simulink model "main_model_mode8"  (R2026a)
settings: Solver=ode4  StopTime=30  FixedStep=1e-4
undefined symbols (not defined in the file or in its folder): dspblkCoreblockFVToolHelper, gcbh
libraries: simulink x12, dspstat3 x3

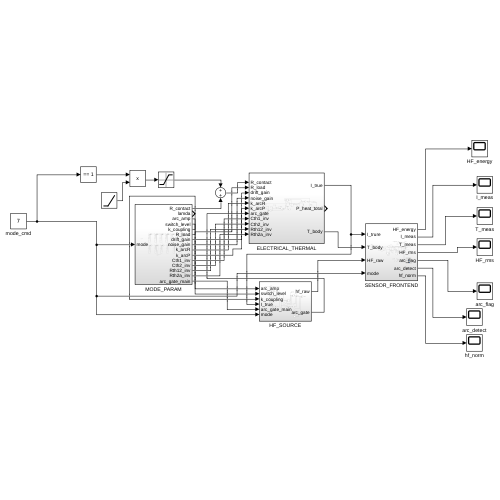
[thumbnail: Simulink's stored preview of the top-level diagram]
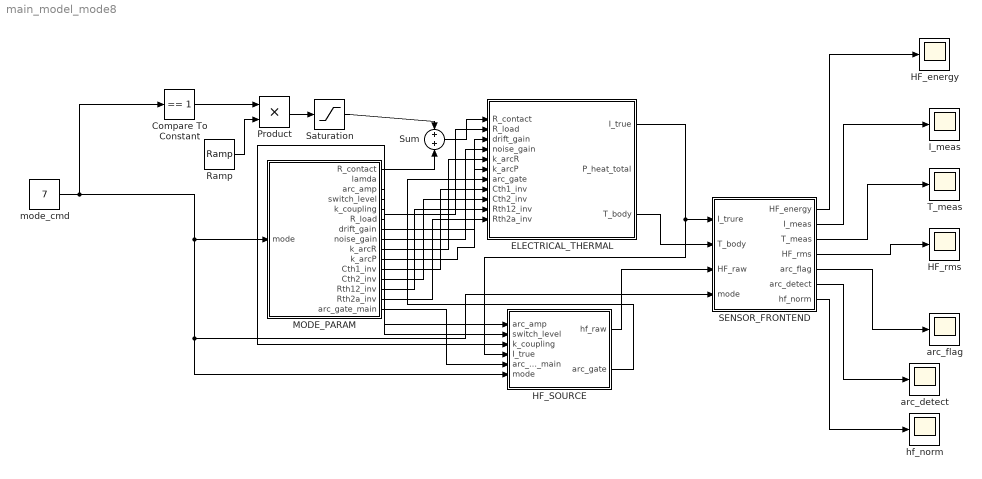
== system main_model_mode8 ==
  Compare To Constant : simulink/Logic and Bit Operations/Compare To Constant  relop===  const=1  OutDataTypeStr=boolean
  ELECTRICAL_THERMAL : Subsystem
  HF_SOURCE : Subsystem
  HF_energy : Scope
      settings: ActiveDisplayYMinimum=-510.38723335588418  ActiveDisplayYMaximum=4593.4851017280953
  HF_rms : Scope
      settings: ActiveDisplayYMinimum=-1  ActiveDisplayYMaximum=1  DataLoggingVariableName=ScopeData3
  I_meas : Scope
      settings: ActiveDisplayYMinimum=-209.09631630294618  ActiveDisplayYMaximum=207.20339945692962
  MODE_PARAM : Subsystem
  Product : Product
  Ramp : simulink/Sources/Ramp  slope=0.002  start=0  InitialOutput=0
  SENSOR_FRONTEND : Subsystem
  Saturation : Saturate  UpperLimit=0.05  LowerLimit=0
  Sum : Sum
  T_meas : Scope
      settings: ActiveDisplayYMinimum=-24.999999999999993  ActiveDisplayYMaximum=225  DataLoggingVariableName=ScopeData2
  arc_detect : Scope
      settings: ActiveDisplayYMinimum=-1  ActiveDisplayYMaximum=1  DataLoggingVariableName=ScopeData10
  arc_flag : Scope
      settings: ActiveDisplayYMinimum=-1  ActiveDisplayYMaximum=1  DataLoggingVariableName=ScopeData9
  hf_norm : Scope
      settings: ActiveDisplayYMinimum=-541.8103571547914  ActiveDisplayYMaximum=4968.8787163023626  DataLoggingVariableName=ScopeData11
  mode_cmd : Constant  Value=7
  wires:
  ELECTRICAL_THERMAL/1(I_true) -> HF_SOURCE/4(I_true), SENSOR_FRONTEND/1(I_trure)
  mode_cmd/1 -> HF_SOURCE/6(mode), SENSOR_FRONTEND/4(mode), MODE_PARAM/1(mode), Compare To Constant/1
  Compare To Constant/1 -> Product/1
  Ramp/1 -> Product/2
  Product/1 -> Saturation/1
  Saturation/1 -> Sum/1
  MODE_PARAM/1(R_contact) -> Sum/2
  Sum/1 -> ELECTRICAL_THERMAL/1(R_contact)
  SENSOR_FRONTEND/2(I_meas) -> I_meas/1
  SENSOR_FRONTEND/3(T_meas) -> T_meas/1
  SENSOR_FRONTEND/1(HF_energy) -> HF_energy/1
  SENSOR_FRONTEND/4(HF_rms) -> HF_rms/1
  MODE_PARAM/6(R_load) -> ELECTRICAL_THERMAL/2(R_load)
  MODE_PARAM/7(drift_gain) -> ELECTRICAL_THERMAL/3(drift_gain)
  MODE_PARAM/8(noise_gain) -> ELECTRICAL_THERMAL/4(noise_gain)
  MODE_PARAM/9(k_arcR) -> ELECTRICAL_THERMAL/5(k_arcR)
  MODE_PARAM/10(k_arcP) -> ELECTRICAL_THERMAL/6(k_arcP)
  MODE_PARAM/11(Cth1_inv) -> ELECTRICAL_THERMAL/8(Cth1_inv)
  MODE_PARAM/12(Cth2_inv) -> ELECTRICAL_THERMAL/9(Cth2_inv)
  MODE_PARAM/13(Rth12_inv) -> ELECTRICAL_THERMAL/10(Rth12_inv)
  MODE_PARAM/14(Rth2a_inv) -> ELECTRICAL_THERMAL/11(Rth2a_inv)
  ELECTRICAL_THERMAL/3(T_body) -> SENSOR_FRONTEND/2(T_body)
  HF_SOURCE/1(hf_raw) -> SENSOR_FRONTEND/3(HF_raw)
  MODE_PARAM/5(k_coupling) -> HF_SOURCE/3(k_coupling)
  MODE_PARAM/4(switch_level) -> HF_SOURCE/2(switch_level)
  MODE_PARAM/3(arc_amp) -> HF_SOURCE/1(arc_amp)
  HF_SOURCE/2(arc_gate) -> ELECTRICAL_THERMAL/7(arc_gate)
  MODE_PARAM/15(arc_gate_main) -> HF_SOURCE/5(arc_gate_main)
  SENSOR_FRONTEND/5(arc_flag) -> arc_flag/1
  SENSOR_FRONTEND/6(arc_detect) -> arc_detect/1
  SENSOR_FRONTEND/7(hf_norm) -> hf_norm/1

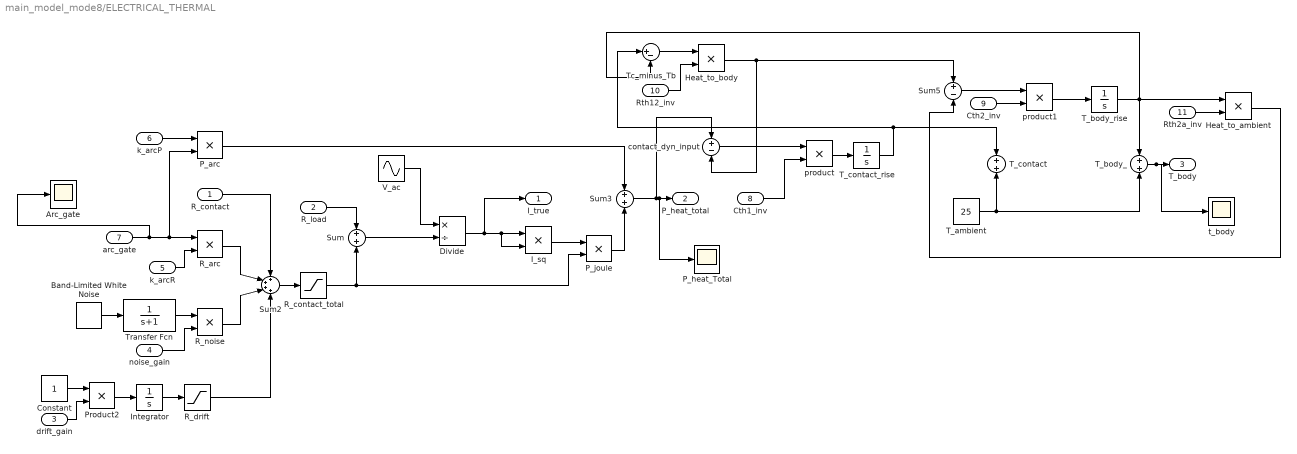
== system main_model_mode8/ELECTRICAL_THERMAL ==
  R_contact : Inport
  R_load : Inport  Port=2
  drift_gain : Inport  Port=3
  noise_gain : Inport  Port=4
  k_arcR : Inport  Port=5
  k_arcP : Inport  Port=6
  arc_gate : Inport  Port=7
  Cth1_inv : Inport  Port=8
  Cth2_inv : Inport  Port=9
  Rth12_inv : Inport  Port=10
  Rth2a_inv : Inport  Port=11
  Arc_gate : Scope
      settings: ActiveDisplayYMinimum=-1  ActiveDisplayYMaximum=1  DataLoggingVariableName=ScopeData5
  Band-Limited White Noise : simulink/Sources/Band-Limited White Noise  Cov=1e-4  Ts=1e-4  seed=11
  Constant : Constant
  Divide : Product  Inputs=*/
  Heat_to_ambient : Product
  Heat_to_body : Product
  I_sq : Product
  Integrator : Integrator
  P_arc : Product
  P_heat_Total : Scope
      settings: ActiveDisplayYMinimum=-108.37902275446248  ActiveDisplayYMaximum=975.41120479016263  DataLoggingVariableName=ScopeData4
  P_joule : Product
  Product2 : Product
  R_arc : Product
  R_contact_total : Saturate  UpperLimit=1  LowerLimit=0.001
  R_drift : Saturate
  R_noise : Product
  Sum : Sum
  Sum2 : Sum  Inputs=++++
  Sum3 : Sum
  Sum5 : Sum  Inputs=+-
  T_ambient : Constant  Value=25
  T_body_ : Sum
  T_body_rise : Integrator
  T_contact : Sum
  T_contact_rise : Integrator
  Tc_minus_Tb : Sum  Inputs=|+-
  Transfer Fcn : TransferFcn  Denominator=[1 1]
  V_ac : Sin  Amplitude=311  Frequency=2*pi*60  SampleTime=1e-4
  contact_dyn_input : Sum  Inputs=+-
  product : Product
  product1 : Product
  t_body : Scope
      settings: ActiveDisplayYMinimum=14.417043129702609  ActiveDisplayYMaximum=120.24661183267655  DataLoggingVariableName=ScopeData7
  I_true : Outport
  P_heat_total : Outport  Port=2
  T_body : Outport  Port=3
  wires:
  R_load/1 -> Sum/1
  Sum/1 -> Divide/2
  V_ac/1 -> Divide/1
  Divide/1 -> I_sq/2, I_sq/1, I_true/1
  I_sq/1 -> P_joule/1
  P_joule/1 -> Sum3/2
  Band-Limited White Noise/1 -> Transfer Fcn/1
  Constant/1 -> Product2/1
  drift_gain/1 -> Product2/2
  Product2/1 -> Integrator/1
  Integrator/1 -> R_drift/1
  Transfer Fcn/1 -> R_noise/1
  noise_gain/1 -> R_noise/2
  arc_gate/1 -> Arc_gate/1, P_arc/2, R_arc/1
  k_arcR/1 -> R_arc/2
  R_contact/1 -> Sum2/1
  R_arc/1 -> Sum2/2
  R_noise/1 -> Sum2/3
  R_drift/1 -> Sum2/4
  Sum2/1 -> R_contact_total/1
  R_contact_total/1 -> P_joule/2, Sum/2
  k_arcP/1 -> P_arc/1
  P_arc/1 -> Sum3/1
  Sum3/1 -> contact_dyn_input/1, P_heat_Total/1, P_heat_total/1
  Tc_minus_Tb/1 -> Heat_to_body/1
  Heat_to_body/1 -> contact_dyn_input/2, Sum5/1
  Cth1_inv/1 -> product/2
  contact_dyn_input/1 -> product/1
  product/1 -> T_contact_rise/1
  T_contact_rise/1 -> T_contact/1, Tc_minus_Tb/1
  Sum5/1 -> product1/1
  Cth2_inv/1 -> product1/2
  product1/1 -> T_body_rise/1
  T_body_rise/1 -> T_body_/1, Heat_to_ambient/1, Tc_minus_Tb/2
  T_ambient/1 -> T_contact/2, T_body_/2
  Rth12_inv/1 -> Heat_to_body/2
  Rth2a_inv/1 -> Heat_to_ambient/2
  Heat_to_ambient/1 -> Sum5/2
  T_body_/1 -> t_body/1, T_body/1

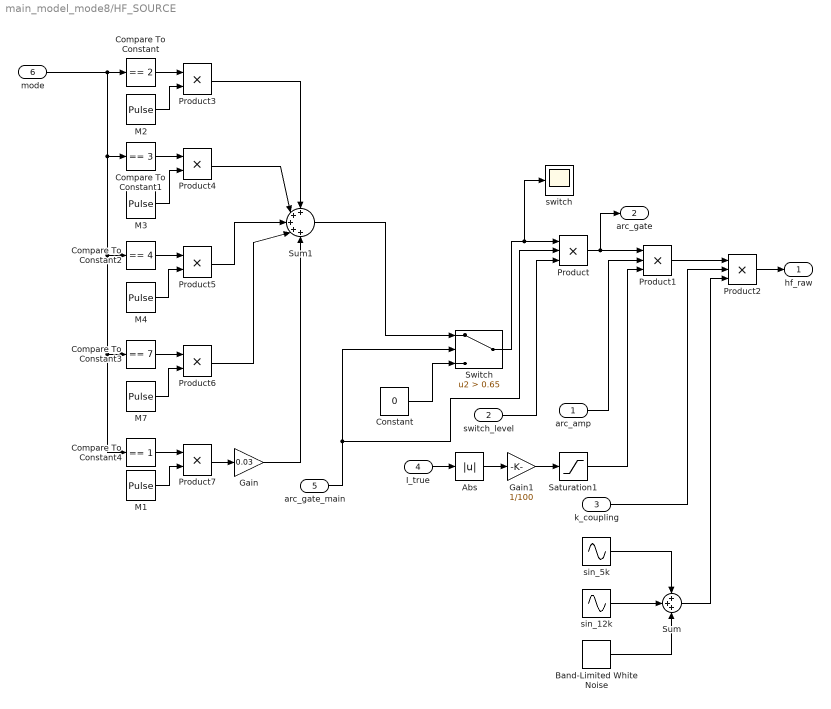
== system main_model_mode8/HF_SOURCE ==
  arc_amp : Inport
  switch_level : Inport  Port=2
  k_coupling : Inport  Port=3
  I_true : Inport  Port=4
  arc_gate_main : Inport  Port=5
  mode : Inport  Port=6
  Abs : Abs  SaturateOnIntegerOverflow=off
  Band-Limited White Noise : simulink/Sources/Band-Limited White Noise  Cov=0.2  Ts=0.0001  seed=[23341]
  Compare To Constant : simulink/Logic and Bit Operations/Compare To Constant  relop===  const=2  OutDataTypeStr=boolean
  Compare To Constant1 : simulink/Logic and Bit Operations/Compare To Constant  relop===  const=3  OutDataTypeStr=boolean
  Compare To Constant2 : simulink/Logic and Bit Operations/Compare To Constant  relop===  const=4  OutDataTypeStr=boolean
  Compare To Constant3 : simulink/Logic and Bit Operations/Compare To Constant  relop===  const=7  OutDataTypeStr=boolean
  Compare To Constant4 : simulink/Logic and Bit Operations/Compare To Constant  relop===  const=1  OutDataTypeStr=boolean
  Constant : Constant  Value=0
  Gain : Gain  Gain=0.03
  Gain1 : Gain  Gain=1/100
  M1 : DiscretePulseGenerator  PulseType=Time based  Amplitude=0.01  Period=0.6  PulseWidth=5
  M2 : DiscretePulseGenerator  PulseType=Time based  Amplitude=0.08  Period=0.4  PulseWidth=10
  M3 : DiscretePulseGenerator  PulseType=Time based  Amplitude=0.25  Period=0.25  PulseWidth=20
  M4 : DiscretePulseGenerator  PulseType=Time based  Amplitude=0.7  Period=0.10  PulseWidth=70
  M7 : DiscretePulseGenerator  PulseType=Time based  Amplitude=0.85  Period=0.08  PulseWidth=80
  Product : Product  Inputs=3
  Product1 : Product  Inputs=3
  Product2 : Product  Inputs=3
  Product{3..7} (5 alike) : Product
  Saturation1 : Saturate  UpperLimit=2.0  LowerLimit=0.5
  Sum : Sum  Inputs=+++
  Sum1 : Sum  Inputs=+++++
  Switch : Switch  Criteria=u2 > Threshold  Threshold=0.65  SaturateOnIntegerOverflow=off  InputSameDT=off
  sin_12k : Sin  Amplitude=0.5  Frequency=2*pi*12000  SampleTime=0.0001
  sin_5k : Sin  Frequency=2*pi*5000  SampleTime=0.0001
  switch : Scope
      settings: ActiveDisplayYMinimum=-0.10624999999999997  ActiveDisplayYMaximum=0.95624999999999993  DataLoggingVariableName=ScopeData8
  hf_raw : Outport
  arc_gate : Outport  Port=2
  wires:
  switch_level/1 -> Product/3
  I_true/1 -> Abs/1
  Abs/1 -> Gain1/1
  Gain1/1 -> Saturation1/1
  Product/1 -> arc_gate/1, Product1/1
  arc_amp/1 -> Product1/2
  Saturation1/1 -> Product1/3
  sin_5k/1 -> Sum/1
  sin_12k/1 -> Sum/2
  Band-Limited White Noise/1 -> Sum/3
  Product1/1 -> Product2/1
  k_coupling/1 -> Product2/2
  Sum/1 -> Product2/3
  Product2/1 -> hf_raw/1
  arc_gate_main/1 -> Switch/2, Product/2
  mode/1 -> Compare To Constant/1, Compare To Constant4/1, Compare To Constant3/1, Compare To Constant2/1, Compare To Constant1/1
  Compare To Constant/1 -> Product3/1
  M2/1 -> Product3/2
  Compare To Constant1/1 -> Product4/1
  M3/1 -> Product4/2
  Compare To Constant2/1 -> Product5/1
  M4/1 -> Product5/2
  Compare To Constant3/1 -> Product6/1
  M7/1 -> Product6/2
  Product3/1 -> Sum1/1
  Product4/1 -> Sum1/2
  Product5/1 -> Sum1/3
  Product6/1 -> Sum1/4
  Constant/1 -> Switch/3
  Switch/1 -> switch/1, Product/1
  Sum1/1 -> Switch/1
  Compare To Constant4/1 -> Product7/1
  M1/1 -> Product7/2
  Product7/1 -> Gain/1
  Gain/1 -> Sum1/5

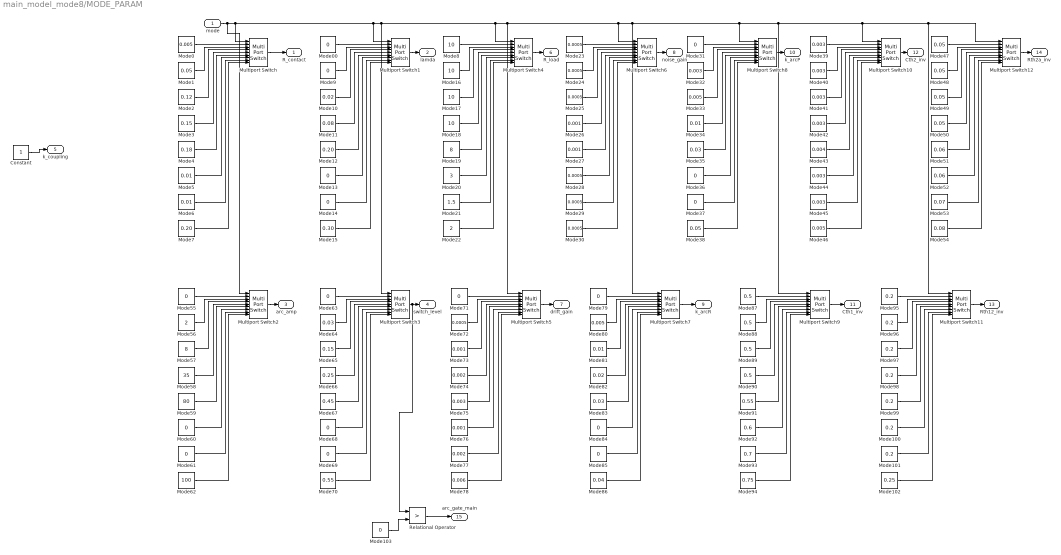
== system main_model_mode8/MODE_PARAM ==
  mode : Inport
  Constant : Constant
  Mode{0,33,46,80} (4 alike) : Constant  Value=0.005
  Mode00 : Constant  Value=0
  Mode{1,38,47..50} (6 alike) : Constant  Value=0.05
  Mode10 : Constant  Value=0.02
  Mode{95..101} (7 alike) : Constant  Value=0.2
  Mode102 : Constant  Value=0.25
  Mode{9,13..14,31,36..37,55,60..61,63,68..69,71,79,84..85,103} (17 alike) : Constant  Value=0
  Mode11 : Constant  Value=0.08
  Mode12 : Constant  Value=0.20
  Mode15 : Constant  Value=0.30
  Mode{8,16..18} (4 alike) : Constant  Value=10
  Mode19 : Constant  Value=8
  Mode2 : Constant  Value=0.12
  Mode20 : Constant  Value=3
  Mode21 : Constant  Value=1.5
  Mode22 : Constant  Value=2
  Mode{23..25,28..30,72} (7 alike) : Constant  Value=0.0005
  Mode{26..27,73,76} (4 alike) : Constant  Value=0.001
  Mode3 : Constant  Value=0.15
  Mode{32,39..42,44..45,75} (8 alike) : Constant  Value=0.003
  Mode{5..6,34,81} (4 alike) : Constant  Value=0.01
  Mode35 : Constant  Value=0.03
  Mode4 : Constant  Value=0.18
  Mode43 : Constant  Value=0.004
  Mode51 : Constant  Value=0.06
  Mode52 : Constant  Value=0.06
  Mode53 : Constant  Value=0.07
  Mode54 : Constant  Value=0.08
  Mode56 : Constant  Value=2
  Mode57 : Constant  Value=8
  Mode58 : Constant  Value=35
  Mode59 : Constant  Value=80
  Mode62 : Constant  Value=100
  Mode64 : Constant  Value=0.03
  Mode65 : Constant  Value=0.15
  Mode66 : Constant  Value=0.25
  Mode67 : Constant  Value=0.45
  Mode7 : Constant  Value=0.20
  Mode70 : Constant  Value=0.55
  Mode74 : Constant  Value=0.002
  Mode77 : Constant  Value=0.002
  Mode78 : Constant  Value=0.006
  Mode82 : Constant  Value=0.02
  Mode83 : Constant  Value=0.03
  Mode86 : Constant  Value=0.04
  Mode{87..90} (4 alike) : Constant  Value=0.5
  Mode91 : Constant  Value=0.55
  Mode92 : Constant  Value=0.6
  Mode93 : Constant  Value=0.7
  Mode94 : Constant  Value=0.75
  Multiport Switch{,1..12} (13 alike) : MultiPortSwitch  DataPortOrder=Zero-based contiguous  Inputs=8  zeroidx=on  SaturateOnIntegerOverflow=off  InputSameDT=off
  Relational Operator : RelationalOperator  Operator=>  OutDataTypeStr=boolean  RndMeth=Simplest  InputSameDT=off
  R_contact : Outport
  lamda : Outport  Port=2
  arc_amp : Outport  Port=3
  switch_level : Outport  Port=4
  k_coupling : Outport  Port=5
  R_load : Outport  Port=6
  drift_gain : Outport  Port=7
  noise_gain : Outport  Port=8
  k_arcR : Outport  Port=9
  k_arcP : Outport  Port=10
  Cth1_inv : Outport  Port=11
  Cth2_inv : Outport  Port=12
  Rth12_inv : Outport  Port=13
  Rth2a_inv : Outport  Port=14
  arc_gate_main : Outport  Port=15
  wires:
  Mode0/1 -> Multiport Switch/2
  Mode1/1 -> Multiport Switch/3
  Mode2/1 -> Multiport Switch/4
  Mode3/1 -> Multiport Switch/5
  mode/1 -> Multiport Switch2/1, Multiport Switch1/1, Multiport Switch3/1, Multiport Switch4/1, Multiport Switch5/1, Multiport Switch6/1, Multiport Switch7/1, Multiport Switch8/1, Multiport Switch9/1, Multiport Switch11/1, Multiport Switch12/1, Multiport Switch10/1, Multiport Switch/1
  Multiport Switch/1 -> R_contact/1
  Constant/1 -> k_coupling/1
  Mode4/1 -> Multiport Switch/6
  Mode5/1 -> Multiport Switch/7
  Mode6/1 -> Multiport Switch/8
  Mode7/1 -> Multiport Switch/9
  Mode12/1 -> Multiport Switch1/6
  Mode13/1 -> Multiport Switch1/7
  Mode15/1 -> Multiport Switch1/9
  Mode9/1 -> Multiport Switch1/3
  Mode14/1 -> Multiport Switch1/8
  Mode00/1 -> Multiport Switch1/2
  Mode11/1 -> Multiport Switch1/5
  Mode10/1 -> Multiport Switch1/4
  Multiport Switch1/1 -> lamda/1
  Mode19/1 -> Multiport Switch4/6
  Mode20/1 -> Multiport Switch4/7
  Mode22/1 -> Multiport Switch4/9
  Mode16/1 -> Multiport Switch4/3
  Mode21/1 -> Multiport Switch4/8
  Mode8/1 -> Multiport Switch4/2
  Mode18/1 -> Multiport Switch4/5
  Mode17/1 -> Multiport Switch4/4
  Multiport Switch4/1 -> R_load/1
  Mode27/1 -> Multiport Switch6/6
  Mode28/1 -> Multiport Switch6/7
  Mode30/1 -> Multiport Switch6/9
  Mode24/1 -> Multiport Switch6/3
  Mode29/1 -> Multiport Switch6/8
  Mode23/1 -> Multiport Switch6/2
  Mode26/1 -> Multiport Switch6/5
  Mode25/1 -> Multiport Switch6/4
  Multiport Switch6/1 -> noise_gain/1
  Mode35/1 -> Multiport Switch8/6
  Mode36/1 -> Multiport Switch8/7
  Mode38/1 -> Multiport Switch8/9
  Mode32/1 -> Multiport Switch8/3
  Mode37/1 -> Multiport Switch8/8
  Mode31/1 -> Multiport Switch8/2
  Mode34/1 -> Multiport Switch8/5
  Mode33/1 -> Multiport Switch8/4
  Multiport Switch8/1 -> k_arcP/1
  Mode43/1 -> Multiport Switch10/6
  Mode44/1 -> Multiport Switch10/7
  Mode46/1 -> Multiport Switch10/9
  Mode40/1 -> Multiport Switch10/3
  Mode45/1 -> Multiport Switch10/8
  Mode39/1 -> Multiport Switch10/2
  Mode42/1 -> Multiport Switch10/5
  Mode41/1 -> Multiport Switch10/4
  Multiport Switch10/1 -> Cth2_inv/1
  Mode51/1 -> Multiport Switch12/6
  Mode52/1 -> Multiport Switch12/7
  Mode54/1 -> Multiport Switch12/9
  Mode48/1 -> Multiport Switch12/3
  Mode53/1 -> Multiport Switch12/8
  Mode47/1 -> Multiport Switch12/2
  Mode50/1 -> Multiport Switch12/5
  Mode49/1 -> Multiport Switch12/4
  Multiport Switch12/1 -> Rth2a_inv/1
  Mode59/1 -> Multiport Switch2/6
  Mode60/1 -> Multiport Switch2/7
  Mode62/1 -> Multiport Switch2/9
  Mode56/1 -> Multiport Switch2/3
  Mode61/1 -> Multiport Switch2/8
  Mode55/1 -> Multiport Switch2/2
  Mode58/1 -> Multiport Switch2/5
  Mode57/1 -> Multiport Switch2/4
  Multiport Switch2/1 -> arc_amp/1
  Mode67/1 -> Multiport Switch3/6
  Mode68/1 -> Multiport Switch3/7
  Mode70/1 -> Multiport Switch3/9
  Mode64/1 -> Multiport Switch3/3
  Mode69/1 -> Multiport Switch3/8
  Mode63/1 -> Multiport Switch3/2
  Mode66/1 -> Multiport Switch3/5
  Mode65/1 -> Multiport Switch3/4
  Multiport Switch3/1 -> Relational Operator/1, switch_level/1
  Mode75/1 -> Multiport Switch5/6
  Mode76/1 -> Multiport Switch5/7
  Mode78/1 -> Multiport Switch5/9
  Mode72/1 -> Multiport Switch5/3
  Mode77/1 -> Multiport Switch5/8
  Mode71/1 -> Multiport Switch5/2
  Mode74/1 -> Multiport Switch5/5
  Mode73/1 -> Multiport Switch5/4
  Multiport Switch5/1 -> drift_gain/1
  Mode83/1 -> Multiport Switch7/6
  Mode84/1 -> Multiport Switch7/7
  Mode86/1 -> Multiport Switch7/9
  Mode80/1 -> Multiport Switch7/3
  Mode85/1 -> Multiport Switch7/8
  Mode79/1 -> Multiport Switch7/2
  Mode82/1 -> Multiport Switch7/5
  Mode81/1 -> Multiport Switch7/4
  Multiport Switch7/1 -> k_arcR/1
  Mode91/1 -> Multiport Switch9/6
  Mode92/1 -> Multiport Switch9/7
  Mode94/1 -> Multiport Switch9/9
  Mode88/1 -> Multiport Switch9/3
  Mode93/1 -> Multiport Switch9/8
  Mode87/1 -> Multiport Switch9/2
  Mode90/1 -> Multiport Switch9/5
  Mode89/1 -> Multiport Switch9/4
  Multiport Switch9/1 -> Cth1_inv/1
  Mode99/1 -> Multiport Switch11/6
  Mode100/1 -> Multiport Switch11/7
  Mode102/1 -> Multiport Switch11/9
  Mode96/1 -> Multiport Switch11/3
  Mode101/1 -> Multiport Switch11/8
  Mode95/1 -> Multiport Switch11/2
  Mode98/1 -> Multiport Switch11/5
  Mode97/1 -> Multiport Switch11/4
  Multiport Switch11/1 -> Rth12_inv/1
  Mode103/1 -> Relational Operator/2
  Relational Operator/1 -> arc_gate_main/1

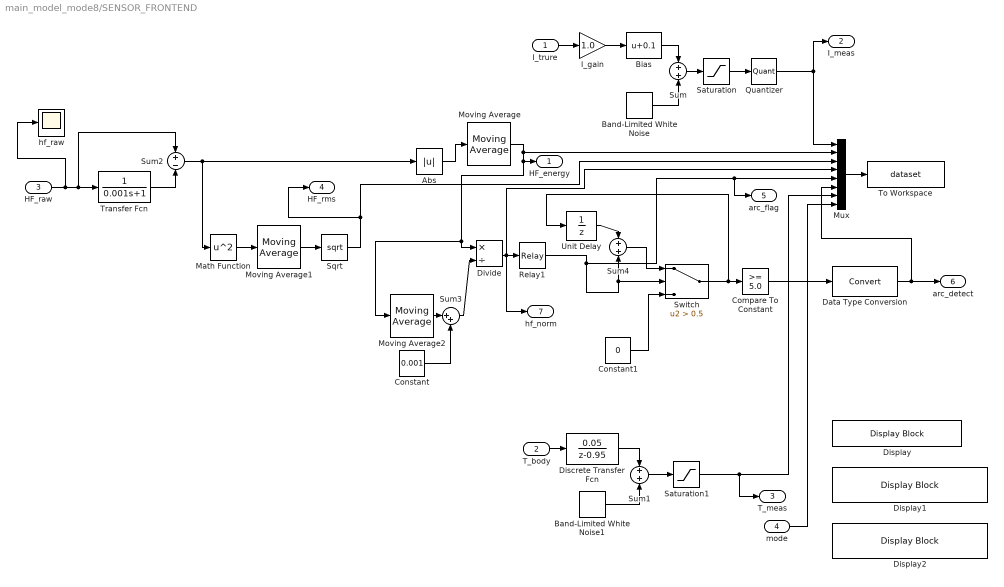
== system main_model_mode8/SENSOR_FRONTEND ==
  I_trure : Inport
  T_body : Inport  Port=2
  HF_raw : Inport  Port=3
  mode : Inport  Port=4
  Abs : Abs  SaturateOnIntegerOverflow=off
  Band-Limited White Noise : simulink/Sources/Band-Limited White Noise  Cov=1e-5  Ts=1e-4  seed=41
  Band-Limited White Noise1 : simulink/Sources/Band-Limited White Noise  Cov=1e-6  Ts=1e-4  seed=51
  Bias : Bias  Bias=0.1  SaturateOnIntegerOverflow=off
  Compare To Constant : simulink/Logic and Bit Operations/Compare To Constant  relop=>=  const=5.0  OutDataTypeStr=boolean
  Constant : Constant  Value=0.001
  Constant1 : Constant  Value=0
  Data Type Conversion : DataTypeConversion  SaturateOnIntegerOverflow=off  RndMeth=Floor
  Discrete Transfer Fcn : DiscreteTransferFcn  LoadFcn=dspblkCoreblockFVToolHelper(gcbh,'load');  Numerator=[0.05]  Denominator=[1 -0.95]
      settings: CopyFcn=dspblkCoreblockFVToolHelper(gcbh,'copy');  DeleteFcn=dspblkCoreblockFVToolHelper(gcbh,'close');  ModelCloseFcn=dspblkCoreblockFVToolHelper(gcbh,'close');  PreSaveFcn=dspblkCoreblockFVToolHelper(gcbh,'presave');  PostSaveFcn=dspblkCoreblockFVToolHelper(gcbh,'postsave');  CloseFcn=dspblkCoreblockFVToolHelper(gcbh,'close');
  Display : DisplayBlock  LabelPosition=Hide  Transparency=1  GridColor=[0.502, 0.502, 0.502]
  Display1 : DisplayBlock  LabelPosition=Hide  Transparency=1  GridColor=[0.502, 0.502, 0.502]
  Display2 : DisplayBlock  LabelPosition=Hide  Transparency=1  GridColor=[0.502, 0.502, 0.502]
  Divide : Product  Inputs=*/
  I_gain : Gain  Gain=1.0
  Math Function : Math  Operator=square
  Moving Average : dspstat3/Moving Average  Method=Sliding window  ForgettingFactorPort=off  SpecifyWindowLength=on  WindowLengthSource=Property  MaxWindowLength=20  WindowLength=50  OverlapLength=49  AllowArbitraryInputLength=off  ForgettingFactor=0.9  SimulateUsing=Interpreted execution
  Moving Average1 : dspstat3/Moving Average  Method=Sliding window  ForgettingFactorPort=off  SpecifyWindowLength=on  WindowLengthSource=Property  MaxWindowLength=20  WindowLength=100  OverlapLength=99  AllowArbitraryInputLength=off  ForgettingFactor=0.9  SimulateUsing=Interpreted execution
  Moving Average2 : dspstat3/Moving Average  Method=Sliding window  ForgettingFactorPort=off  SpecifyWindowLength=on  WindowLengthSource=Property  MaxWindowLength=20  WindowLength=1000  OverlapLength=999  AllowArbitraryInputLength=off  ForgettingFactor=0.9  SimulateUsing=Interpreted execution
  Mux : Mux  Inputs=8
  Quantizer : Quantizer  QuantizationInterval=0.1
  Relay1 : Relay  OnSwitchValue=0.05  OffSwitchValue=0.03
  Saturation : Saturate  UpperLimit=300  LowerLimit=-300
  Saturation1 : Saturate  UpperLimit=200  LowerLimit=0
  Sqrt : Sqrt
  Sum : Sum
  Sum1 : Sum
  Sum2 : Sum  Inputs=+-
  Sum3 : Sum  Inputs=|++
  Sum4 : Sum
  Switch : Switch  Criteria=u2 > Threshold  Threshold=0.5  SaturateOnIntegerOverflow=off  InputSameDT=off
  To Workspace : ToWorkspace  VariableName=dataset  SampleTime=-1
  Transfer Fcn : TransferFcn  Denominator=[0.001 1]
  Unit Delay : UnitDelay  SampleTime=-1
  hf_raw : Scope
      settings: ActiveDisplayYMinimum=-14433.49218432861  ActiveDisplayYMaximum=14666.347077384213  DataLoggingVariableName=ScopeData6
  HF_energy : Outport
  I_meas : Outport  Port=2
  T_meas : Outport  Port=3
  HF_rms : Outport  Port=4
  arc_flag : Outport  Port=5
  arc_detect : Outport  Port=6
  hf_norm : Outport  Port=7
  wires:
  Abs/1 -> Moving Average/1
  Moving Average/1 -> Divide/1, Moving Average2/1, HF_energy/1, Mux/2
  I_trure/1 -> I_gain/1
  Band-Limited White Noise/1 -> Sum/2
  Band-Limited White Noise1/1 -> Sum1/2
  Mux/1 -> To Workspace/1
  Saturation/1 -> Quantizer/1
  I_gain/1 -> Bias/1
  Bias/1 -> Sum/1
  Sum/1 -> Saturation/1
  Quantizer/1 -> I_meas/1, Mux/1
  Saturation1/1 -> Mux/7, T_meas/1
  Sum1/1 -> Saturation1/1
  Moving Average1/1 -> Sqrt/1
  Sum2/1 -> Abs/1, Math Function/1
  Math Function/1 -> Moving Average1/1
  T_body/1 -> Discrete Transfer Fcn/1
  Discrete Transfer Fcn/1 -> Sum1/1
  HF_raw/1 -> hf_raw/1, Sum2/1, Transfer Fcn/1
  Transfer Fcn/1 -> Sum2/2
  Sqrt/1 -> HF_rms/1, Mux/3
  Moving Average2/1 -> Sum3/1
  Constant/1 -> Sum3/2
  Sum3/1 -> Divide/2
  Divide/1 -> hf_norm/1, Mux/4, Relay1/1
  Constant1/1 -> Switch/3
  Sum4/1 -> Switch/1
  Unit Delay/1 -> Sum4/1
  Relay1/1 -> arc_flag/1, Mux/5, Switch/2, Sum4/2
  Switch/1 -> Compare To Constant/1, Unit Delay/1
  mode/1 -> Mux/8
  Compare To Constant/1 -> Data Type Conversion/1
  Data Type Conversion/1 -> Mux/6, arc_detect/1
